simulink library "GyroscopeProcessing_lib"  (R2018b)
settings: Solver=VariableStepAuto  StartTime=0.0  StopTime=10.0  RelTol=1e-3
undefined symbols (not defined in the file or in its folder): fswParams, u1, u2, u3
libraries: dspindex x18, simulink x9, two_norm x9
settings Model: Creator=sophiakim  LastModifiedBy=Nick's PC

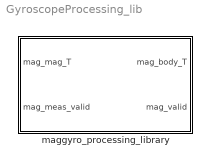
== system GyroscopeProcessing_lib ==
  maggyro_processing_library : Subsystem  mask{static_range_max_value=fswParams.sensors.gyro_static_range, rotation_calibration_matrix1=fswParams.sensors.gyro_rotate1, rotation_calibration_matrix2=fswParams.sensors.gyro_rotate2, rotation_calibration_matrix3=fswParams.sensors.gyro_rotate3, offset_calibration_matrix=fswParams.sensors.gyro_offset, mag_max_err=fswParams.sensors.gyro_max_err}
      mask prompts: static_range_max_value "Max Static Range"; rotation_calibration_matrix1 "Rotation Calibration Matrix 1"; rotation_calibration_matrix2 "Rotation Calibration Matrix 2"; rotation_calibration_matrix3 "Rotation Calibration Matrix 3"; offset_calibration_matrix "Offset Calibration Matrix"; mag_max_err "Max Error Allowed"
      mask TypeOptions static_range_max_value:
      | Static Range Check
      | /Check
      | Static Range1/max | Static Range Check
      | /Check
      | Static Range2/max | Static Range Check
      | /Check
      | Static Range4/max
      mask TypeOptions rotation_calibration_matrix1: Body Frame Converter/mag_rotate1/Value
      mask TypeOptions rotation_calibration_matrix2: Body Frame Converter/mag_rotate2/Value
      mask TypeOptions rotation_calibration_matrix3: Body Frame Converter/mag_rotate3/Value
      mask TypeOptions offset_calibration_matrix: Body Frame Converter/mag_offset/Value
      mask TypeOptions mag_max_err:
      | If Action
      | Subsystem 3/Compare
      | To Constant/const | If Action
      | Subsystem 3/Compare
      | To Constant1/const | If Action
      | Subsystem 3/Compare
      | To Constant2/const | If Action
      | Subsystem 2/If Action
      | Subsystem1/Compare
      | To Constant/const | If Action
      | Subsystem 2/If Action
      | Subsystem14/Compare
      | To Constant/const | If Action
      | Subsystem 2/If Action
      | Subsystem2/Compare
      | To Constant/const

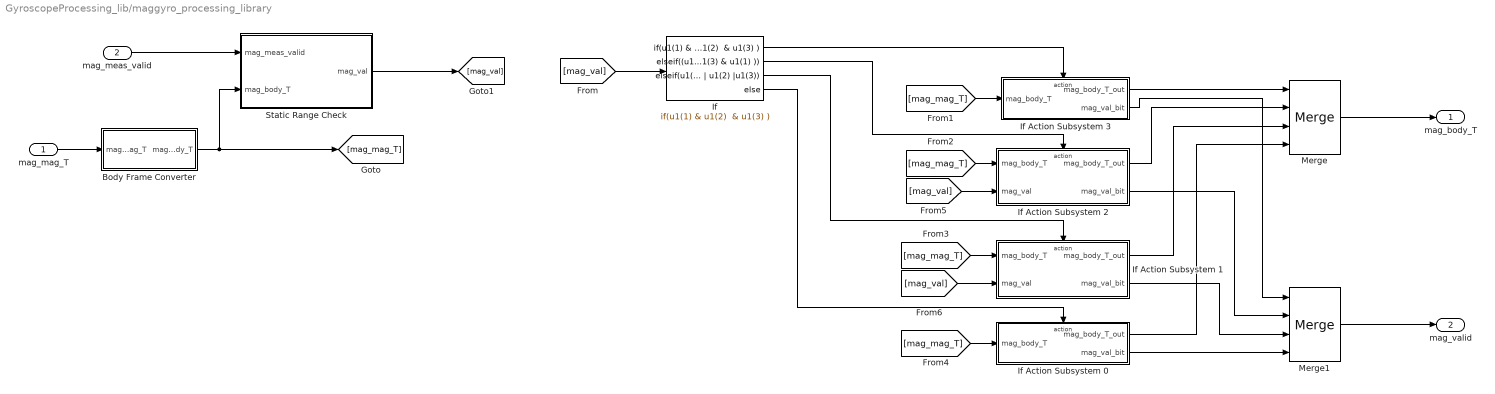
== system GyroscopeProcessing_lib/maggyro_processing_library ==
  mag_mag_T : Inport
  mag_meas_valid : Inport  Port=2
  Body Frame Converter : Subsystem
  If : If  IfExpression="u1(1) & u1(2)  & u1(3)"  ElseIfExpressions=(u1(1) & u1(2) ) | (u1(2) & u1(3) )|(u1(3) & u1(1) ), u1(1) | u1(2) |u1(3)
  If Action Subsystem 0 : Subsystem  TreatAsAtomicUnit=on
  If Action Subsystem 1 : Subsystem  TreatAsAtomicUnit=on
  If Action Subsystem 2 : Subsystem  TreatAsAtomicUnit=on
  If Action Subsystem 3 : Subsystem  TreatAsAtomicUnit=on
  Merge : Merge  Inputs=4
  Merge1 : Merge  Inputs=4
  "Static Range Check " : Subsystem
  mag_body_T : Outport
  mag_valid : Outport  Port=2
  wires:
  "Static Range Check "/1(mag_val) -> [mag_val]
  If Action Subsystem 3/1(mag_body_T_out) -> Merge/1
  If Action Subsystem 0/2(mag_val_bit) -> Merge1/4
  If/4 -> If Action Subsystem 0/Action
  [mag_val] -> If/1
  [mag_mag_T] -> If Action Subsystem 1/1(mag_body_T)
  [mag_val] -> If Action Subsystem 1/2(mag_val)
  If Action Subsystem 1/1(mag_body_T_out) -> Merge/3
  If Action Subsystem 2/2(mag_val_bit) -> Merge1/2
  If Action Subsystem 0/1(mag_body_T_out) -> Merge/4
  [mag_mag_T] -> If Action Subsystem 2/1(mag_body_T)
  If/1 -> If Action Subsystem 3/Action
  If Action Subsystem 3/2(mag_val_bit) -> Merge1/1
  If/2 -> If Action Subsystem 2/Action
  If/3 -> If Action Subsystem 1/Action
  If Action Subsystem 1/2(mag_val_bit) -> Merge1/3
  If Action Subsystem 2/1(mag_body_T_out) -> Merge/2
  [mag_mag_T] -> If Action Subsystem 3/1(mag_body_T)
  [mag_mag_T] -> If Action Subsystem 0/1(mag_body_T)
  [mag_val] -> If Action Subsystem 2/2(mag_val)
  Merge/1 -> mag_body_T/1
  Merge1/1 -> mag_valid/1
  mag_meas_valid/1 -> "Static Range Check "/1(mag_meas_valid)
  mag_mag_T/1 -> Body Frame Converter/1(mag_mag_T)
  Body Frame Converter/1(mag_body_T) -> [mag_mag_T], "Static Range Check "/2(mag_body_T)

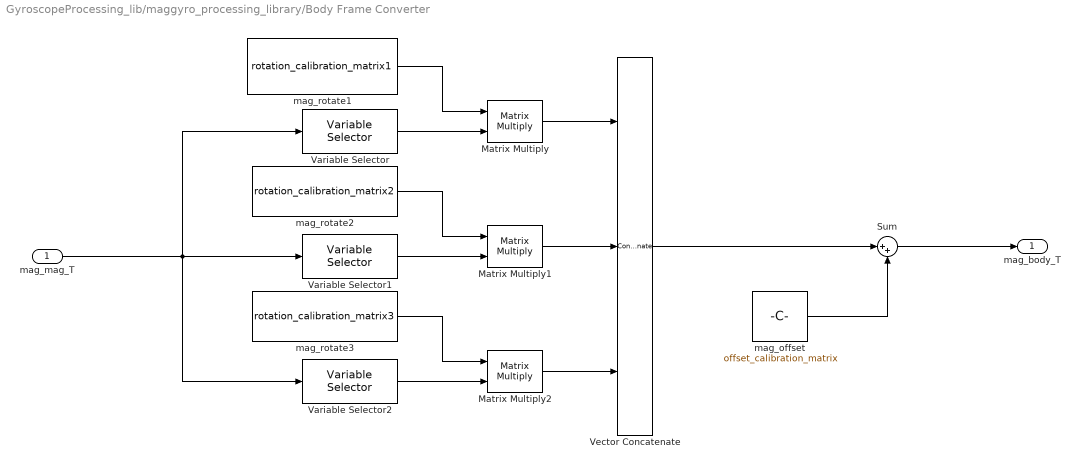
== system GyroscopeProcessing_lib/maggyro_processing_library/Body Frame Converter ==
  mag_mag_T : Inport
  Matrix Multiply : Product  Multiplication=Matrix(*)
  Matrix Multiply1 : Product  Multiplication=Matrix(*)
  Matrix Multiply2 : Product  Multiplication=Matrix(*)
  Sum : Sum  Inputs=|++
  Variable Selector : dspindex/Variable Selector  NumInputs=1  rowsOrCols=Columns  IdxMode=Fixed  Elements=[1]  ZerOneIdxMode=One-based  errmode=Clip Index  FillMode=on  FillValues=0
  Variable Selector1 : dspindex/Variable Selector  NumInputs=1  rowsOrCols=Columns  IdxMode=Fixed  Elements=[2]  ZerOneIdxMode=One-based  errmode=Clip Index  FillMode=on  FillValues=0
  Variable Selector2 : dspindex/Variable Selector  NumInputs=1  rowsOrCols=Columns  IdxMode=Fixed  Elements=[3]  ZerOneIdxMode=One-based  errmode=Clip Index  FillMode=on  FillValues=0
  Vector Concatenate : Concatenate  NumInputs=3  Mode=Multidimensional array  ConcatenateDimension=2
  mag_offset : Constant  Value=offset_calibration_matrix
  mag_rotate1 : Constant  Value=rotation_calibration_matrix1
  mag_rotate2 : Constant  Value=rotation_calibration_matrix2
  mag_rotate3 : Constant  Value=rotation_calibration_matrix3
  mag_body_T : Outport
  wires:
  mag_offset/1 -> Sum/2
  Sum/1 -> mag_body_T/1
  mag_mag_T/1 -> Variable Selector/1, Variable Selector2/1, Variable Selector1/1
  Variable Selector/1 -> Matrix Multiply/2
  mag_rotate1/1 -> Matrix Multiply/1
  Variable Selector1/1 -> Matrix Multiply1/2
  Variable Selector2/1 -> Matrix Multiply2/2
  mag_rotate2/1 -> Matrix Multiply1/1
  mag_rotate3/1 -> Matrix Multiply2/1
  Matrix Multiply/1 -> Vector Concatenate/1
  Matrix Multiply1/1 -> Vector Concatenate/2
  Matrix Multiply2/1 -> Vector Concatenate/3
  Vector Concatenate/1 -> Sum/1

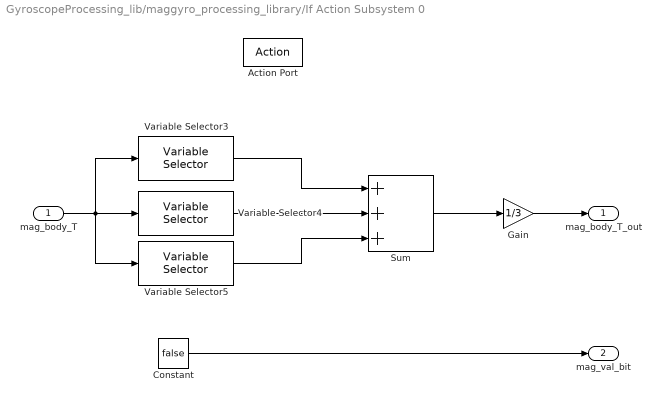
== system GyroscopeProcessing_lib/maggyro_processing_library/If Action Subsystem 0 ==
  mag_body_T : Inport
  Action Port : ActionPort  ActionType=else
  Constant : Constant  Value=false
  Gain : Gain  Gain=1/3
  Sum : Sum  Inputs=+++
  Variable Selector3 : dspindex/Variable Selector  NumInputs=1  rowsOrCols=Columns  IdxMode=Fixed  Elements=[1]  ZerOneIdxMode=One-based  errmode=Clip Index  FillMode=on  FillValues=0
  Variable Selector4 : dspindex/Variable Selector  NumInputs=1  rowsOrCols=Columns  IdxMode=Fixed  Elements=[2]  ZerOneIdxMode=One-based  errmode=Clip Index  FillMode=on  FillValues=0
  Variable Selector5 : dspindex/Variable Selector  NumInputs=1  rowsOrCols=Columns  IdxMode=Fixed  Elements=[3]  ZerOneIdxMode=One-based  errmode=Clip Index  FillMode=on  FillValues=0
  mag_body_T_out : Outport
  mag_val_bit : Outport  Port=2
  wires:
  Sum/1 -> Gain/1
  Variable Selector5/1 -> Sum/3
  Variable Selector4/1 -> Sum/2
  Variable Selector3/1 -> Sum/1
  mag_body_T/1 -> Variable Selector5/1, Variable Selector3/1, Variable Selector4/1
  Gain/1 -> mag_body_T_out/1
  Constant/1 -> mag_val_bit/1

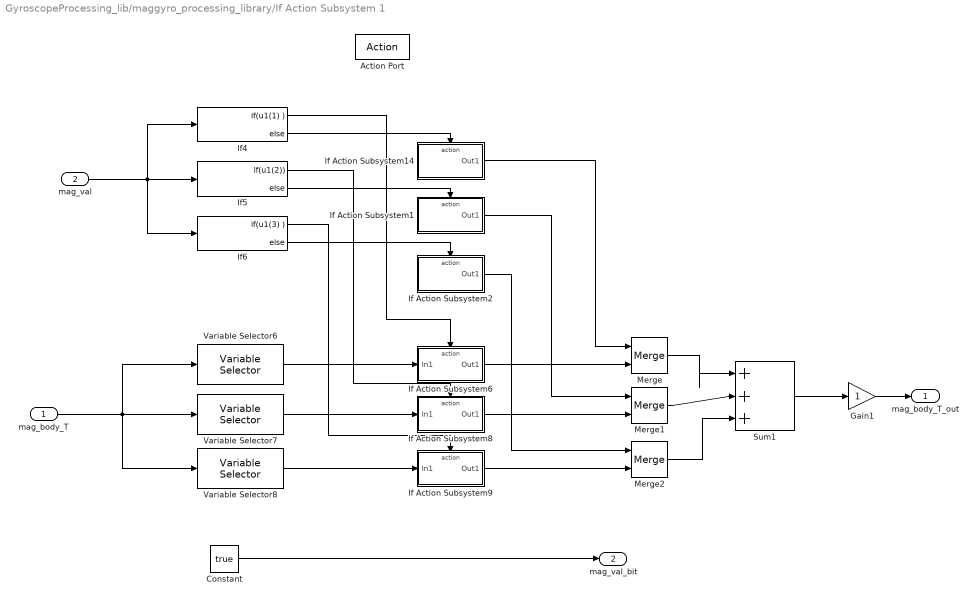
== system GyroscopeProcessing_lib/maggyro_processing_library/If Action Subsystem 1 ==
  mag_body_T : Inport
  mag_val : Inport  Port=2
  Action Port : ActionPort  ActionType=elseif
  Constant : Constant  Value=true
  Gain1 : Gain
  If Action Subsystem1 : Subsystem  TreatAsAtomicUnit=on
  If Action Subsystem14 : Subsystem  TreatAsAtomicUnit=on
  If Action Subsystem2 : Subsystem  TreatAsAtomicUnit=on
  If Action Subsystem6 : Subsystem  TreatAsAtomicUnit=on
  If Action Subsystem8 : Subsystem  TreatAsAtomicUnit=on
  If Action Subsystem9 : Subsystem  TreatAsAtomicUnit=on
  If4 : If  IfExpression=u1(1)
  If5 : If  IfExpression=u1(2)
  If6 : If  IfExpression=u1(3)
  Merge : Merge
  Merge1 : Merge
  Merge2 : Merge
  Sum1 : Sum  Inputs=|+++
  Variable Selector6 : dspindex/Variable Selector  NumInputs=1  rowsOrCols=Columns  IdxMode=Fixed  Elements=[1]  ZerOneIdxMode=One-based  errmode=Clip Index  FillMode=on  FillValues=0
  Variable Selector7 : dspindex/Variable Selector  NumInputs=1  rowsOrCols=Columns  IdxMode=Fixed  Elements=[2]  ZerOneIdxMode=One-based  errmode=Clip Index  FillMode=on  FillValues=0
  Variable Selector8 : dspindex/Variable Selector  NumInputs=1  rowsOrCols=Columns  IdxMode=Fixed  Elements=[3]  ZerOneIdxMode=One-based  errmode=Clip Index  FillMode=on  FillValues=0
  mag_body_T_out : Outport
  mag_val_bit : Outport  Port=2
  wires:
  Gain1/1 -> mag_body_T_out/1
  If Action Subsystem6/1(Out1) -> Merge/2
  If4/2 -> If Action Subsystem14/Action
  If6/1 -> If Action Subsystem9/Action
  Sum1/1 -> Gain1/1
  If4/1 -> If Action Subsystem6/Action
  Variable Selector8/1 -> If Action Subsystem9/1(In1)
  Variable Selector6/1 -> If Action Subsystem6/1(In1)
  If Action Subsystem1/1(Out1) -> Merge1/1
  If5/1 -> If Action Subsystem8/Action
  Merge/1 -> Sum1/1
  If Action Subsystem9/1(Out1) -> Merge2/2
  If Action Subsystem2/1(Out1) -> Merge2/1
  Merge2/1 -> Sum1/3
  If Action Subsystem8/1(Out1) -> Merge1/2
  Variable Selector7/1 -> If Action Subsystem8/1(In1)
  Merge1/1 -> Sum1/2
  If6/2 -> If Action Subsystem2/Action
  If Action Subsystem14/1(Out1) -> Merge/1
  If5/2 -> If Action Subsystem1/Action
  mag_body_T/1 -> Variable Selector6/1, Variable Selector8/1, Variable Selector7/1
  mag_val/1 -> If6/1, If4/1, If5/1
  Constant/1 -> mag_val_bit/1

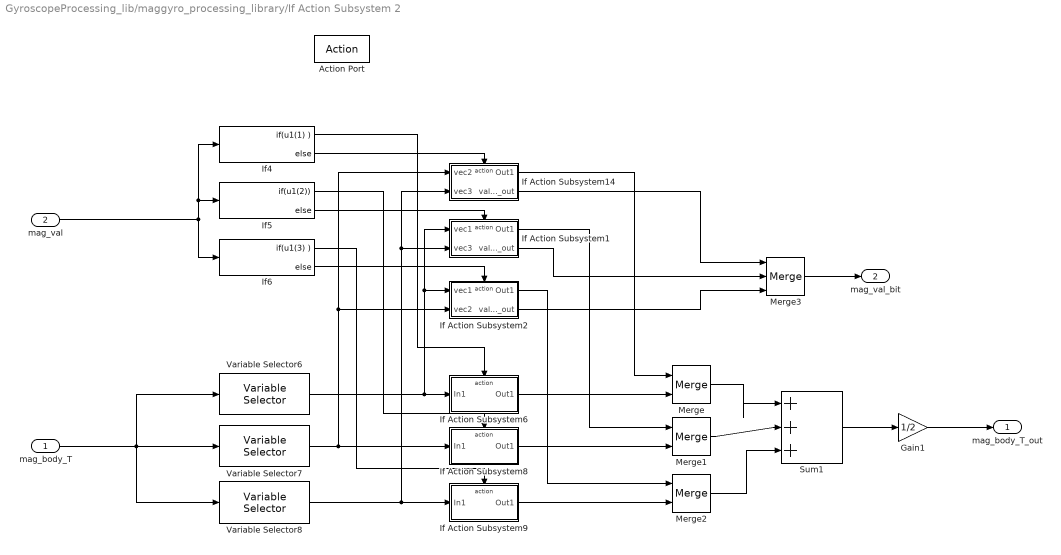
== system GyroscopeProcessing_lib/maggyro_processing_library/If Action Subsystem 2 ==
  mag_body_T : Inport
  mag_val : Inport  Port=2
  Action Port : ActionPort  ActionType=elseif
  Gain1 : Gain  Gain=1/2
  If Action Subsystem1 : Subsystem  TreatAsAtomicUnit=on
  If Action Subsystem14 : Subsystem  TreatAsAtomicUnit=on
  If Action Subsystem2 : Subsystem  TreatAsAtomicUnit=on
  If Action Subsystem6 : Subsystem  TreatAsAtomicUnit=on
  If Action Subsystem8 : Subsystem  TreatAsAtomicUnit=on
  If Action Subsystem9 : Subsystem  TreatAsAtomicUnit=on
  If4 : If  IfExpression=u1(1)
  If5 : If  IfExpression=u1(2)
  If6 : If  IfExpression=u1(3)
  Merge : Merge
  Merge1 : Merge
  Merge2 : Merge
  Merge3 : Merge  Inputs=3
  Sum1 : Sum  Inputs=|+++
  Variable Selector6 : dspindex/Variable Selector  NumInputs=1  rowsOrCols=Columns  IdxMode=Fixed  Elements=[1]  ZerOneIdxMode=One-based  errmode=Clip Index  FillMode=on  FillValues=0
  Variable Selector7 : dspindex/Variable Selector  NumInputs=1  rowsOrCols=Columns  IdxMode=Fixed  Elements=[2]  ZerOneIdxMode=One-based  errmode=Clip Index  FillMode=on  FillValues=0
  Variable Selector8 : dspindex/Variable Selector  NumInputs=1  rowsOrCols=Columns  IdxMode=Fixed  Elements=[3]  ZerOneIdxMode=One-based  errmode=Clip Index  FillMode=on  FillValues=0
  mag_body_T_out : Outport
  mag_val_bit : Outport  Port=2
  wires:
  Variable Selector7/1 -> If Action Subsystem2/2(vec2), If Action Subsystem14/1(vec2), If Action Subsystem8/1(In1)
  mag_val/1 -> If4/1, If5/1, If6/1
  If5/1 -> If Action Subsystem8/Action
  If6/1 -> If Action Subsystem9/Action
  If4/1 -> If Action Subsystem6/Action
  Variable Selector6/1 -> If Action Subsystem2/1(vec1), If Action Subsystem1/1(vec1), If Action Subsystem6/1(In1)
  Variable Selector8/1 -> If Action Subsystem1/2(vec3), If Action Subsystem14/2(vec3), If Action Subsystem9/1(In1)
  Gain1/1 -> mag_body_T_out/1
  Sum1/1 -> Gain1/1
  mag_body_T/1 -> Variable Selector8/1, Variable Selector7/1, Variable Selector6/1
  If4/2 -> If Action Subsystem14/Action
  If Action Subsystem14/1(Out1) -> Merge/1
  If Action Subsystem6/1(Out1) -> Merge/2
  Merge/1 -> Sum1/1
  If Action Subsystem8/1(Out1) -> Merge1/2
  If Action Subsystem9/1(Out1) -> Merge2/2
  Merge2/1 -> Sum1/3
  Merge1/1 -> Sum1/2
  If5/2 -> If Action Subsystem1/Action
  If6/2 -> If Action Subsystem2/Action
  If Action Subsystem1/1(Out1) -> Merge1/1
  If Action Subsystem2/1(Out1) -> Merge2/1
  If Action Subsystem14/2(valid_out) -> Merge3/1
  If Action Subsystem1/2(valid_out) -> Merge3/2
  If Action Subsystem2/2(valid_out) -> Merge3/3
  Merge3/1 -> mag_val_bit/1

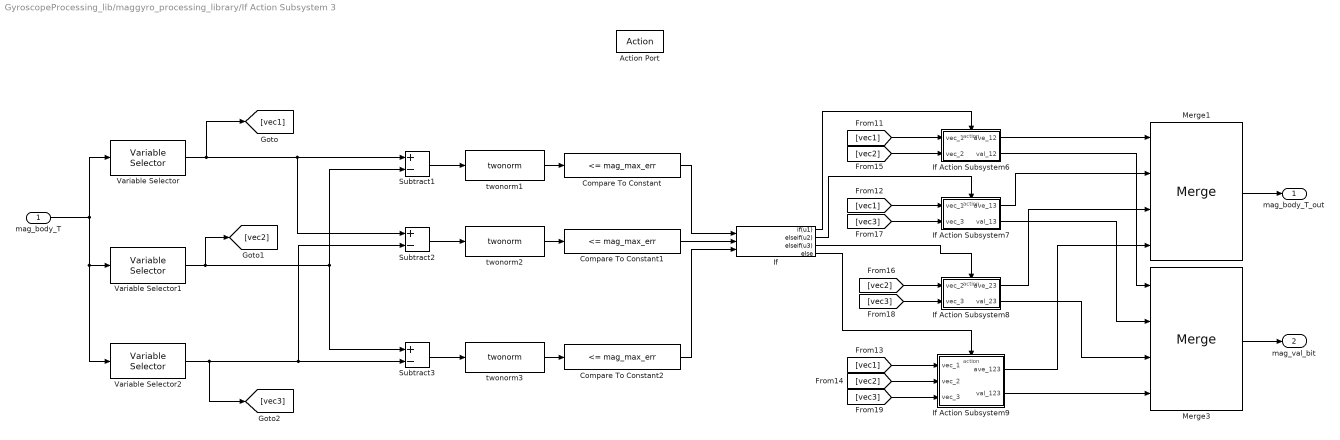
== system GyroscopeProcessing_lib/maggyro_processing_library/If Action Subsystem 3 ==
  mag_body_T : Inport
  Action Port : ActionPort  ActionType=then
  Compare To Constant : simulink/Logic and Bit Operations/Compare To Constant  relop=<=  const=mag_max_err  OutDataTypeStr=boolean
  Compare To Constant1 : simulink/Logic and Bit Operations/Compare To Constant  relop=<=  const=mag_max_err  OutDataTypeStr=boolean
  Compare To Constant2 : simulink/Logic and Bit Operations/Compare To Constant  relop=<=  const=mag_max_err  OutDataTypeStr=boolean
  If : If  NumInputs=3  IfExpression=u1  ElseIfExpressions=u2,u3
  If Action Subsystem6 : Subsystem  TreatAsAtomicUnit=on
  If Action Subsystem7 : Subsystem  TreatAsAtomicUnit=on
  If Action Subsystem8 : Subsystem  TreatAsAtomicUnit=on
  If Action Subsystem9 : Subsystem  TreatAsAtomicUnit=on
  Merge1 : Merge  Inputs=4
  Merge3 : Merge  Inputs=4
  Subtract1 : Sum  Inputs=+-
  Subtract2 : Sum  Inputs=+-
  Subtract3 : Sum  Inputs=+-
  Variable Selector : dspindex/Variable Selector  NumInputs=1  rowsOrCols=Columns  IdxMode=Fixed  Elements=[1]  ZerOneIdxMode=One-based  errmode=Clip Index  FillMode=on  FillValues=0
  Variable Selector1 : dspindex/Variable Selector  NumInputs=1  rowsOrCols=Columns  IdxMode=Fixed  Elements=[2]  ZerOneIdxMode=One-based  errmode=Clip Index  FillMode=on  FillValues=0
  Variable Selector2 : dspindex/Variable Selector  NumInputs=1  rowsOrCols=Columns  IdxMode=Fixed  Elements=[3]  ZerOneIdxMode=One-based  errmode=Clip Index  FillMode=on  FillValues=0
  twonorm1 : two_norm/twonorm  SystemSampleTime=-1
  twonorm2 : two_norm/twonorm  SystemSampleTime=-1
  twonorm3 : two_norm/twonorm  SystemSampleTime=-1
  mag_body_T_out : Outport
  mag_val_bit : Outport  Port=2
  wires:
  mag_body_T/1 -> Variable Selector1/1, Variable Selector2/1, Variable Selector/1
  Variable Selector/1 -> Subtract2/1, Subtract1/1, [vec1]
  If Action Subsystem6/1(ave_12) -> Merge1/1
  If Action Subsystem7/1(ave_13) -> Merge1/2
  If Action Subsystem8/1(ave_23) -> Merge1/3
  If Action Subsystem9/1(ave_123) -> Merge1/4
  If Action Subsystem6/2(val_12) -> Merge3/1
  If Action Subsystem7/2(val_13) -> Merge3/2
  If Action Subsystem8/2(val_23) -> Merge3/3
  If Action Subsystem9/2(val_123) -> Merge3/4
  Variable Selector1/1 -> [vec2], Subtract3/1, Subtract1/2
  Variable Selector2/1 -> Subtract2/2, Subtract3/2, [vec3]
  Subtract3/1 -> twonorm3/1
  Subtract2/1 -> twonorm2/1
  Subtract1/1 -> twonorm1/1
  If/1 -> If Action Subsystem6/Action
  If/2 -> If Action Subsystem7/Action
  If/3 -> If Action Subsystem8/Action
  If/4 -> If Action Subsystem9/Action
  [vec1] -> If Action Subsystem6/1(vec_1)
  [vec1] -> If Action Subsystem7/1(vec_1)
  [vec1] -> If Action Subsystem9/1(vec_1)
  [vec2] -> If Action Subsystem9/2(vec_2)
  [vec2] -> If Action Subsystem6/2(vec_2)
  [vec2] -> If Action Subsystem8/1(vec_2)
  [vec3] -> If Action Subsystem7/2(vec_3)
  [vec3] -> If Action Subsystem8/2(vec_3)
  [vec3] -> If Action Subsystem9/3(vec_3)
  Merge1/1 -> mag_body_T_out/1
  Merge3/1 -> mag_val_bit/1
  Compare To Constant/1 -> If/1
  twonorm1/1 -> Compare To Constant/1
  twonorm2/1 -> Compare To Constant1/1
  Compare To Constant1/1 -> If/2
  twonorm3/1 -> Compare To Constant2/1
  Compare To Constant2/1 -> If/3

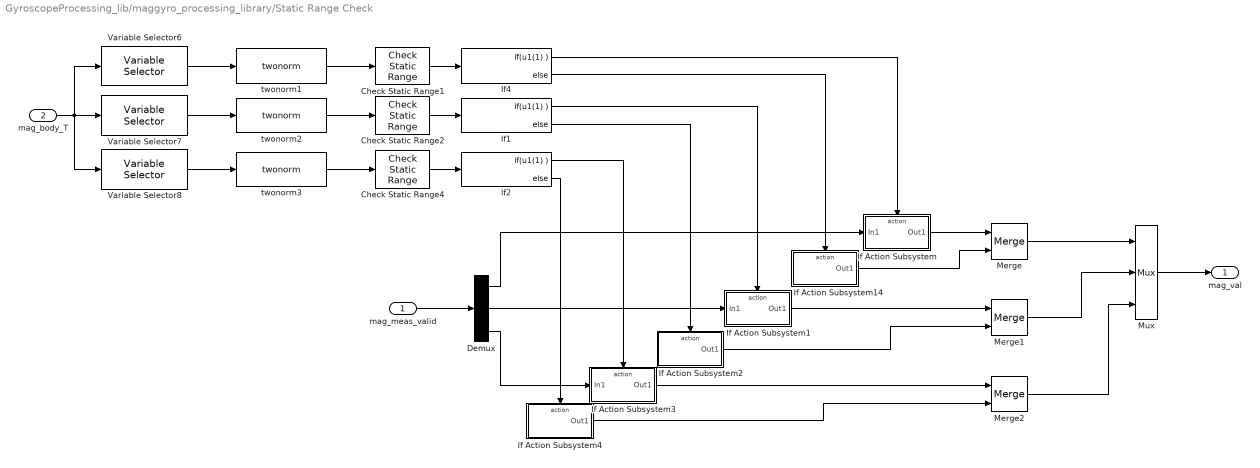
== system GyroscopeProcessing_lib/maggyro_processing_library/Static Range Check  ==
  mag_meas_valid : Inport
  mag_body_T : Inport  Port=2
  Check Static Range1 : simulink/Model Verification/Check  Static Range  Description=0 <= u <= static_range_max_value  max=static_range_max_value  max_included=on  min=0  min_included=on  enabled=on  stopWhenAssertionFail=off  export=on  icon=graphic
      settings: SourceProductName=Simulink  SourceProductBaseCode=SL
  Check Static Range2 : simulink/Model Verification/Check  Static Range  Description=0 <= u <= static_range_max_value  max=static_range_max_value  max_included=on  min=0  min_included=on  enabled=on  stopWhenAssertionFail=off  export=on  icon=graphic
      settings: SourceProductName=Simulink  SourceProductBaseCode=SL
  Check Static Range4 : simulink/Model Verification/Check  Static Range  Description=0 <= u <= static_range_max_value  max=static_range_max_value  max_included=on  min=0  min_included=on  enabled=on  stopWhenAssertionFail=off  export=on  icon=graphic
      settings: SourceProductName=Simulink  SourceProductBaseCode=SL
  Demux : Demux  Outputs=3
  If Action Subsystem : Subsystem  TreatAsAtomicUnit=on
  If Action Subsystem1 : Subsystem  TreatAsAtomicUnit=on
  If Action Subsystem14 : Subsystem  TreatAsAtomicUnit=on
  If Action Subsystem2 : Subsystem  TreatAsAtomicUnit=on
  If Action Subsystem3 : Subsystem  TreatAsAtomicUnit=on
  If Action Subsystem4 : Subsystem  TreatAsAtomicUnit=on
  If1 : If  IfExpression=u1(1)
  If2 : If  IfExpression=u1(1)
  If4 : If  IfExpression=u1(1)
  Merge : Merge
  Merge1 : Merge
  Merge2 : Merge
  Mux : Mux  Inputs=3
  Variable Selector6 : dspindex/Variable Selector  NumInputs=1  rowsOrCols=Columns  IdxMode=Fixed  Elements=[1]  ZerOneIdxMode=One-based  errmode=Clip Index  FillMode=on  FillValues=0
  Variable Selector7 : dspindex/Variable Selector  NumInputs=1  rowsOrCols=Columns  IdxMode=Fixed  Elements=[2]  ZerOneIdxMode=One-based  errmode=Clip Index  FillMode=on  FillValues=0
  Variable Selector8 : dspindex/Variable Selector  NumInputs=1  rowsOrCols=Columns  IdxMode=Fixed  Elements=[3]  ZerOneIdxMode=One-based  errmode=Clip Index  FillMode=on  FillValues=0
  twonorm1 : two_norm/twonorm  SystemSampleTime=-1
  twonorm2 : two_norm/twonorm  SystemSampleTime=-1
  twonorm3 : two_norm/twonorm  SystemSampleTime=-1
  mag_val : Outport
  wires:
  If2/2 -> If Action Subsystem4/Action
  If2/1 -> If Action Subsystem3/Action
  If4/2 -> If Action Subsystem14/Action
  Check Static Range1/1 -> If4/1
  If4/1 -> If Action Subsystem/Action
  Check Static Range4/1 -> If2/1
  If1/2 -> If Action Subsystem2/Action
  Demux/1 -> If Action Subsystem/1(In1)
  If1/1 -> If Action Subsystem1/Action
  If Action Subsystem/1(Out1) -> Merge/1
  If Action Subsystem14/1(Out1) -> Merge/2
  If Action Subsystem1/1(Out1) -> Merge1/1
  If Action Subsystem2/1(Out1) -> Merge1/2
  If Action Subsystem3/1(Out1) -> Merge2/1
  If Action Subsystem4/1(Out1) -> Merge2/2
  Demux/3 -> If Action Subsystem3/1(In1)
  Merge/1 -> Mux/1
  Merge1/1 -> Mux/2
  Merge2/1 -> Mux/3
  Mux/1 -> mag_val/1
  mag_body_T/1 -> Variable Selector8/1, Variable Selector7/1, Variable Selector6/1
  Check Static Range2/1 -> If1/1
  Variable Selector6/1 -> twonorm1/1
  Variable Selector8/1 -> twonorm3/1
  mag_meas_valid/1 -> Demux/1
  Demux/2 -> If Action Subsystem1/1(In1)
  twonorm1/1 -> Check Static Range1/1
  twonorm2/1 -> Check Static Range2/1
  twonorm3/1 -> Check Static Range4/1
  Variable Selector7/1 -> twonorm2/1

== system GyroscopeProcessing_lib/maggyro_processing_library/If Action Subsystem 1/If Action Subsystem1 ==
  Action Port : ActionPort
  Constant : Constant  Value=[0;0;0]
  Out1 : Outport
  wires:
  Constant/1 -> Out1/1

== system GyroscopeProcessing_lib/maggyro_processing_library/If Action Subsystem 1/If Action Subsystem14 ==
  Action Port : ActionPort
  Constant : Constant  Value=[0;0;0]
  Out1 : Outport
  wires:
  Constant/1 -> Out1/1

== system GyroscopeProcessing_lib/maggyro_processing_library/If Action Subsystem 1/If Action Subsystem2 ==
  Action Port : ActionPort
  Constant : Constant  Value=[0;0;0]
  Out1 : Outport
  wires:
  Constant/1 -> Out1/1

== system GyroscopeProcessing_lib/maggyro_processing_library/If Action Subsystem 1/If Action Subsystem6 ==
  In1 : Inport
  Action Port : ActionPort
  Out1 : Outport
  wires:
  In1/1 -> Out1/1

== system GyroscopeProcessing_lib/maggyro_processing_library/If Action Subsystem 1/If Action Subsystem8 ==
  In1 : Inport
  Action Port : ActionPort
  Out1 : Outport
  wires:
  In1/1 -> Out1/1

== system GyroscopeProcessing_lib/maggyro_processing_library/If Action Subsystem 1/If Action Subsystem9 ==
  In1 : Inport
  Action Port : ActionPort
  Out1 : Outport
  wires:
  In1/1 -> Out1/1

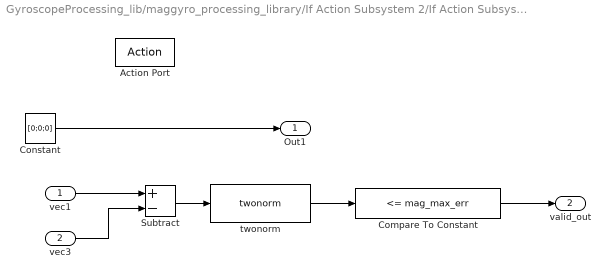
== system GyroscopeProcessing_lib/maggyro_processing_library/If Action Subsystem 2/If Action Subsystem1 ==
  vec1 : Inport
  vec3 : Inport  Port=2
  Action Port : ActionPort
  Compare To Constant : simulink/Logic and Bit Operations/Compare To Constant  relop=<=  const=mag_max_err  OutDataTypeStr=boolean
  Constant : Constant  Value=[0;0;0]
  Subtract : Sum  Inputs=+-
  twonorm : two_norm/twonorm  SystemSampleTime=-1
  Out1 : Outport
  valid_out : Outport  Port=2
  wires:
  Constant/1 -> Out1/1
  Subtract/1 -> twonorm/1
  vec1/1 -> Subtract/1
  vec3/1 -> Subtract/2
  Compare To Constant/1 -> valid_out/1
  twonorm/1 -> Compare To Constant/1

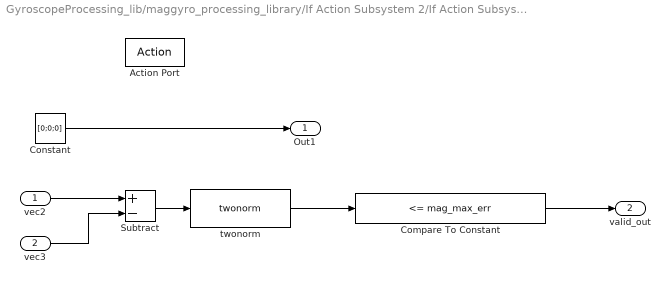
== system GyroscopeProcessing_lib/maggyro_processing_library/If Action Subsystem 2/If Action Subsystem14 ==
  vec2 : Inport
  vec3 : Inport  Port=2
  Action Port : ActionPort
  Compare To Constant : simulink/Logic and Bit Operations/Compare To Constant  relop=<=  const=mag_max_err  OutDataTypeStr=boolean
  Constant : Constant  Value=[0;0;0]
  Subtract : Sum  Inputs=+-
  twonorm : two_norm/twonorm  SystemSampleTime=-1
  Out1 : Outport
  valid_out : Outport  Port=2
  wires:
  Constant/1 -> Out1/1
  vec2/1 -> Subtract/1
  vec3/1 -> Subtract/2
  Subtract/1 -> twonorm/1
  Compare To Constant/1 -> valid_out/1
  twonorm/1 -> Compare To Constant/1

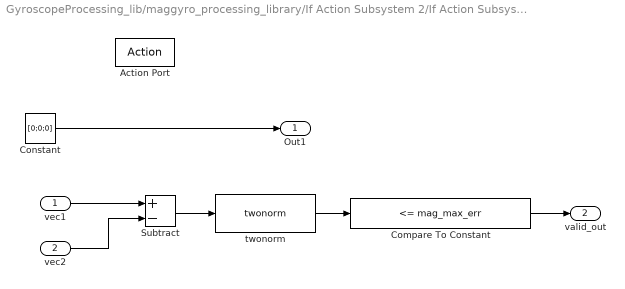
== system GyroscopeProcessing_lib/maggyro_processing_library/If Action Subsystem 2/If Action Subsystem2 ==
  vec1 : Inport
  vec2 : Inport  Port=2
  Action Port : ActionPort
  Compare To Constant : simulink/Logic and Bit Operations/Compare To Constant  relop=<=  const=mag_max_err  OutDataTypeStr=boolean
  Constant : Constant  Value=[0;0;0]
  Subtract : Sum  Inputs=+-
  twonorm : two_norm/twonorm  SystemSampleTime=-1
  Out1 : Outport
  valid_out : Outport  Port=2
  wires:
  Constant/1 -> Out1/1
  Subtract/1 -> twonorm/1
  vec1/1 -> Subtract/1
  vec2/1 -> Subtract/2
  Compare To Constant/1 -> valid_out/1
  twonorm/1 -> Compare To Constant/1

== system GyroscopeProcessing_lib/maggyro_processing_library/If Action Subsystem 2/If Action Subsystem6 ==
  In1 : Inport
  Action Port : ActionPort
  Out1 : Outport
  wires:
  In1/1 -> Out1/1

== system GyroscopeProcessing_lib/maggyro_processing_library/If Action Subsystem 2/If Action Subsystem8 ==
  In1 : Inport
  Action Port : ActionPort
  Out1 : Outport
  wires:
  In1/1 -> Out1/1

== system GyroscopeProcessing_lib/maggyro_processing_library/If Action Subsystem 2/If Action Subsystem9 ==
  In1 : Inport
  Action Port : ActionPort
  Out1 : Outport
  wires:
  In1/1 -> Out1/1

== system GyroscopeProcessing_lib/maggyro_processing_library/If Action Subsystem 3/If Action Subsystem6 ==
  vec_1 : Inport
  vec_2 : Inport  Port=2
  Action Port : ActionPort  ActionType=then
  Constant : Constant  Value=true
  Gain : Gain  Gain=1/2
  Sum : Sum  Inputs=|++
  ave_12 : Outport
  val_12 : Outport  Port=2
  wires:
  vec_1/1 -> Sum/1
  vec_2/1 -> Sum/2
  Sum/1 -> Gain/1
  Gain/1 -> ave_12/1
  Constant/1 -> val_12/1

== system GyroscopeProcessing_lib/maggyro_processing_library/If Action Subsystem 3/If Action Subsystem7 ==
  vec_1 : Inport
  vec_3 : Inport  Port=2
  Action Port : ActionPort  ActionType=elseif
  Constant : Constant  Value=true
  Gain : Gain  Gain=1/2
  Sum : Sum  Inputs=|++
  ave_13 : Outport
  val_13 : Outport  Port=2
  wires:
  vec_1/1 -> Sum/1
  vec_3/1 -> Sum/2
  Constant/1 -> val_13/1
  Sum/1 -> Gain/1
  Gain/1 -> ave_13/1

== system GyroscopeProcessing_lib/maggyro_processing_library/If Action Subsystem 3/If Action Subsystem8 ==
  vec_2 : Inport
  vec_3 : Inport  Port=2
  Action Port : ActionPort  ActionType=elseif
  Constant : Constant  Value=true
  Gain : Gain  Gain=1/2
  Sum : Sum  Inputs=|++
  ave_23 : Outport
  val_23 : Outport  Port=2
  wires:
  vec_2/1 -> Sum/1
  vec_3/1 -> Sum/2
  Constant/1 -> val_23/1
  Sum/1 -> Gain/1
  Gain/1 -> ave_23/1

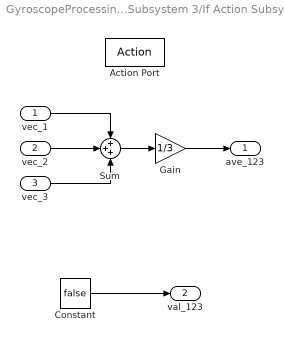
== system GyroscopeProcessing_lib/maggyro_processing_library/If Action Subsystem 3/If Action Subsystem9 ==
  vec_1 : Inport
  vec_2 : Inport  Port=2
  vec_3 : Inport  Port=3
  Action Port : ActionPort  ActionType=else
  Constant : Constant  Value=false
  Gain : Gain  Gain=1/3
  Sum : Sum  Inputs=+++
  ave_123 : Outport
  val_123 : Outport  Port=2
  wires:
  vec_1/1 -> Sum/1
  vec_2/1 -> Sum/2
  Constant/1 -> val_123/1
  Sum/1 -> Gain/1
  Gain/1 -> ave_123/1
  vec_3/1 -> Sum/3

== system GyroscopeProcessing_lib/maggyro_processing_library/Static Range Check /If Action Subsystem ==
  In1 : Inport
  Action Port : ActionPort
  Out1 : Outport
  wires:
  In1/1 -> Out1/1

== system GyroscopeProcessing_lib/maggyro_processing_library/Static Range Check /If Action Subsystem1 ==
  In1 : Inport
  Action Port : ActionPort
  Out1 : Outport
  wires:
  In1/1 -> Out1/1

== system GyroscopeProcessing_lib/maggyro_processing_library/Static Range Check /If Action Subsystem14 ==
  Action Port : ActionPort
  Constant : Constant  Value=0  OutDataTypeStr=boolean
  Out1 : Outport
  wires:
  Constant/1 -> Out1/1

== system GyroscopeProcessing_lib/maggyro_processing_library/Static Range Check /If Action Subsystem2 ==
  Action Port : ActionPort
  Constant : Constant  Value=0  OutDataTypeStr=boolean
  Out1 : Outport
  wires:
  Constant/1 -> Out1/1

== system GyroscopeProcessing_lib/maggyro_processing_library/Static Range Check /If Action Subsystem3 ==
  In1 : Inport
  Action Port : ActionPort
  Out1 : Outport
  wires:
  In1/1 -> Out1/1

== system GyroscopeProcessing_lib/maggyro_processing_library/Static Range Check /If Action Subsystem4 ==
  Action Port : ActionPort
  Constant : Constant  Value=0  OutDataTypeStr=boolean
  Out1 : Outport
  wires:
  Constant/1 -> Out1/1
